simulink model "problema2"  (R2021a)
settings: Solver=VariableStepAuto  StartTime=0.0  StopTime=100  RelTol=1e-3
settings Model: Creator=Usuario  LastModifiedBy=Usuario
settings DataIOCC: ReturnWorkspaceOutputs=off

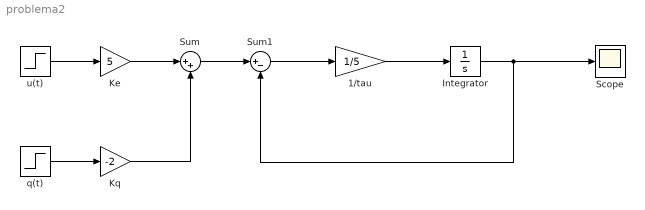
== system problema2 ==
  1/tau : Gain  Gain=1/5
  Integrator : Integrator
  Ke : Gain  Gain=5
  Kq : Gain  Gain=-2
  Scope : Scope
  Sum : Sum  Inputs=|++
  Sum1 : Sum  Inputs=|+-
  q(t) : Step  Time=50  SampleTime=0
  u(t) : Step  Time=10  SampleTime=0
  wires:
  u(t)/1 -> Ke/1
  q(t)/1 -> Kq/1
  Ke/1 -> Sum/1
  Sum1/1 -> 1/tau/1
  1/tau/1 -> Integrator/1
  Integrator/1 -> Scope/1, Sum1/2
  Kq/1 -> Sum/2
  Sum/1 -> Sum1/1
